simulink subsystem "PID_discreto"  (R2023b)
settings: Solver=VariableStepAuto  StartTime=0.0  StopTime=10.0  RelTol=1e-3
values from neighbouring files (symbols this model uses):
  b_a = 0.0396    [parametros.m]
  k_sa = 31.656    [parametros.m]
  k_sia = 10130    [parametros.m]
settings Model: Creator=nicol  LastModifiedBy=nicol

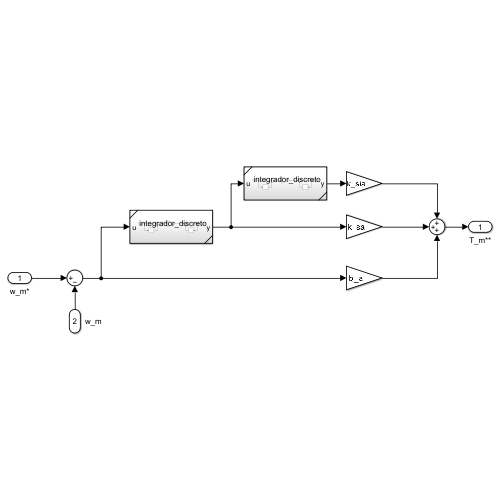
[thumbnail: Simulink's stored preview of the top-level diagram]
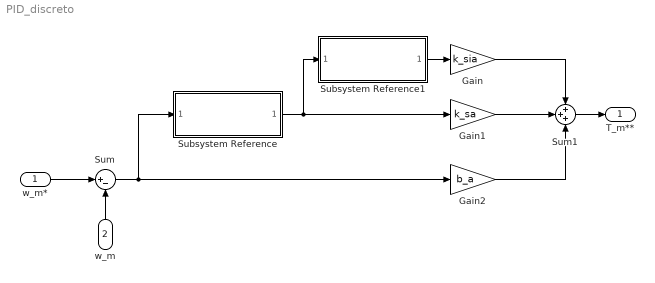
== system PID_discreto ==
  w_m* : Inport
  w_m : Inport  Port=2
  Gain : Gain  Gain=k_sia
  Gain1 : Gain  Gain=k_sa
  Gain2 : Gain  Gain=b_a
  Subsystem Reference : Subsystem  ReferencedSubsystem=integrador_discreto
  Subsystem Reference1 : Subsystem  ReferencedSubsystem=integrador_discreto
  Sum : Sum  Inputs=|+-
  Sum1 : Sum  Inputs=+++
  T_m** : Outport
  wires:
  Gain1/1 -> Sum1/2
  Sum1/1 -> T_m**/1
  Gain/1 -> Sum1/1
  Gain2/1 -> Sum1/3
  w_m/1 -> Sum/2
  Sum/1 -> Subsystem Reference/1, Gain2/1
  w_m*/1 -> Sum/1
  Subsystem Reference/1 -> Subsystem Reference1/1, Gain1/1
  Subsystem Reference1/1 -> Gain/1
